simulink model "my_block_diagram"  (R2018a)
settings: Solver=VariableStepAuto  StartTime=0.0  StopTime=1.49  RelTol=1e-3
values from neighbouring files (symbols this model uses):
  A_d = eye(ns)+dt*[0 0 1 0 0 0;0 0 0 1 0 0;0 0 -k 0 1 0;0 0 0 -k 0 1;0 0 0 0 -1/tau 0; 0 0 0 0 0 -1/tau]    [my_controller.m]
  B_d = zeros(ns,nu); B_d(5,1) = dt/tau; B_d(6,2) = dt/tau    [my_controller.m]
  C_d = diag([1 1 1 1 1 1])    [my_controller.m]
  D_d = zeros(ns, nu)    [my_controller.m]
  delay = 10    [my_controller.m]
  dt = 0.01    [my_controller.m]
  L_k = zeros(N,nu,ns)    [my_controller.m]
  ns = 6    [my_controller.m]
  nu = 2    [my_controller.m]
  x_init = [0.1;0.1;0;0;0;0]    [my_controller.m]
libraries: cstblocks x1
settings Model: PauseTimes=50  Creator=tomek  LastModifiedBy=tomek

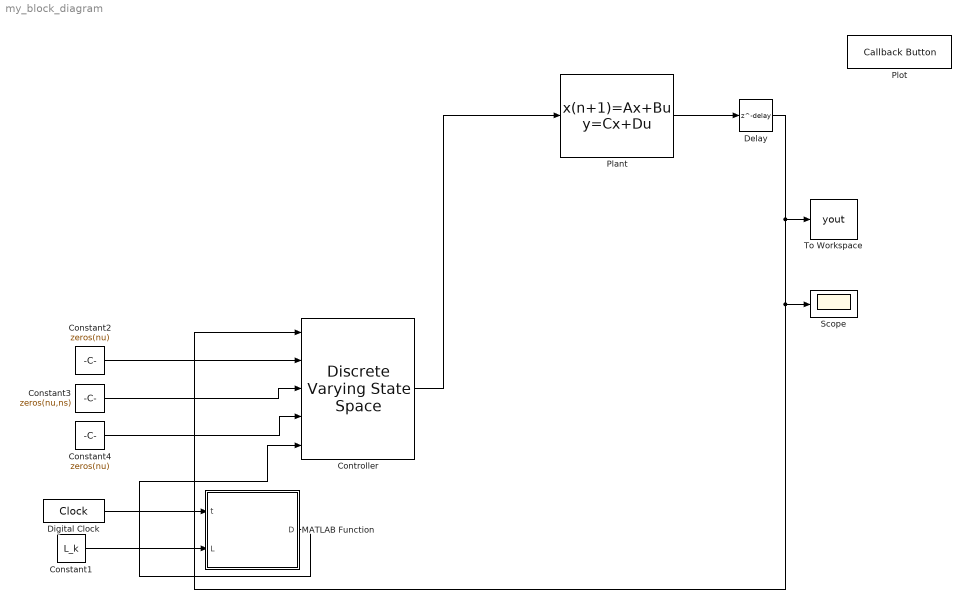
== system my_block_diagram ==
  Constant1 : Constant  Value=L_k
  Constant2 : Constant  Value=zeros(nu)  SampleTime=dt
  Constant3 : Constant  Value=zeros(nu,ns)  SampleTime=dt
  Constant4 : Constant  Value=zeros(nu)  SampleTime=dt
  "Controller " : cstblocks/Linear Parameter Varying/Discrete Varying State Space  x0=0  Ts=dt  OutputX=off  OutputDX=off
      settings: SourceProductName=Control System Toolbox  SourceProductBaseCode=CT
  Delay : Delay  DelayLength=delay  InitialCondition=repmat(x_init, 1, delay)  InputProcessing=Inherited  SampleTime=dt
  Digital Clock : DigitalClock  SampleTime=dt
  MATLAB Function : MATLAB Function  TreatAsAtomicUnit=on
  "Plant " : DiscreteStateSpace  A=A_d  B=B_d  C=C_d  D=D_d  InitialCondition=x_init  SampleTime=dt
  Plot : CallbackButton  WebBlockId=47  ButtonText=Plot results
      settings: ClickFcn=|
      | subplot(2,2,1);
      | plot(dt*linspace(0,1.5,N),yout(:,1))
      | subplot(2,2,2);
      | plot(dt*linspace(0,1.5,N),yout(:,2))
      | subplot(2,2,3);
      | plot(dt*linspace(0,1.5,N),yout(:,3))
      | subplot(2,2,4);
      | plot(dt*linspace(0,1.5,N),yout(:,4))
  Scope : Scope
  To Workspace : ToWorkspace  VariableName=yout  SampleTime=-1
      settings: Save2DSignal=2-D array (concatenate along first dimension)
  wires:
  Digital Clock/1 -> MATLAB Function/1(t)
  Constant1/1 -> MATLAB Function/2(L)
  MATLAB Function/1(D) -> "Controller "/5
  Constant4/1 -> "Controller "/4
  Constant3/1 -> "Controller "/3
  Constant2/1 -> "Controller "/2
  "Controller "/1 -> "Plant "/1
  "Plant "/1 -> Delay/1
  Delay/1 -> To Workspace/1, Scope/1, "Controller "/1

== matlab function my_block_diagram/MATLAB Function ==
  data: t input; D output; L input
function D = fcn(t, L)

index = t+0.01;
index = round(index/0.01);
D = -squeeze(L(index,:,:));
